simulink model "Kalman_validation"  (R2019a)
settings: Solver=VariableStepAuto  StartTime=0.0  StopTime=100.0  RelTol=1e-3
undefined symbols (not defined in the file or in its folder): DiscIntNeverNeededParam, Discrete, Time
libraries: simulink x3, ctrlSharedLib x2
settings Model: Creator=Gaming  LastModifiedBy=Gaming

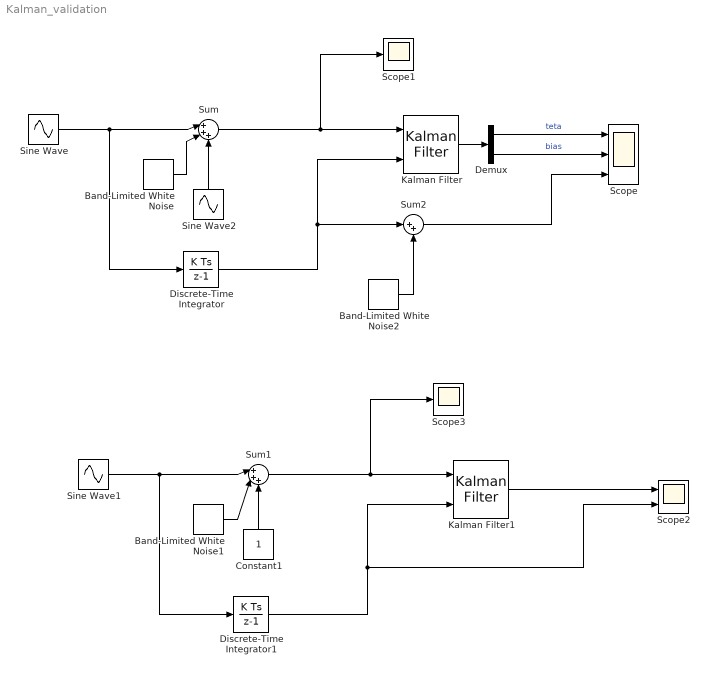
== system Kalman_validation ==
  Band-Limited White Noise : simulink/Sources/Band-Limited White Noise  Cov=[0.0001]  Ts=0.1  seed=[23341]
  Band-Limited White Noise1 : simulink/Sources/Band-Limited White Noise  Cov=[0.0001]  Ts=0.1  seed=[23341]
  Band-Limited White Noise2 : simulink/Sources/Band-Limited White Noise  Cov=[0.0001]  Ts=0.1  seed=[23341]
  Constant1 : Constant
  Demux : Demux  Outputs=2
  Discrete-Time Integrator : DiscreteIntegrator  SampleTime=-1  ICPrevOutput=DiscIntNeverNeededParam  ICPrevScaledInput=DiscIntNeverNeededParam
  Discrete-Time Integrator1 : DiscreteIntegrator  SampleTime=-1  ICPrevOutput=DiscIntNeverNeededParam  ICPrevScaledInput=DiscIntNeverNeededParam
  Kalman Filter : ctrlSharedLib/Kalman Filter  TimeDomain=Discrete-Time  UseCurrentEstimator=on  ModelSource=LTI State-Space Variable  ModelSourceVariable=ALFA  A=0.95*eye(2)  B=eye(2)  C=eye(2)  D=zeros(2)  NumberOfStates=2  NumberOfInputs=2  NumberOfOutputs=2  InitialEstimateSource=Dialog  X0=[0,;0]  P0=10  UseK=off  UseGH=off  NumberOfProcessNoiseInputs=2  G=1  TimeInvariantG=on  H=0  TimeInvariantH=on  Q=1000  TimeInvariantQ=on  R=1  TimeInvariantR=on  N=0  TimeInvariantN=on  AddInputPort=on  AddEnablePort=off  OutputEstimatedY=off  OutputP=off  Ts=-1
      settings: SourceProductBaseCode=CT
  Kalman Filter1 : ctrlSharedLib/Kalman Filter  TimeDomain=Discrete-Time  UseCurrentEstimator=on  ModelSource=LTI State-Space Variable  ModelSourceVariable=BETA  A=0.95*eye(2)  B=eye(2)  C=eye(2)  D=zeros(2)  NumberOfStates=2  NumberOfInputs=2  NumberOfOutputs=2  InitialEstimateSource=Dialog  X0=0  P0=10  UseK=off  UseGH=off  NumberOfProcessNoiseInputs=2  G=1  TimeInvariantG=on  H=0  TimeInvariantH=on  Q=1000  TimeInvariantQ=on  R=1  TimeInvariantR=on  N=0  TimeInvariantN=on  AddInputPort=on  AddEnablePort=off  OutputEstimatedY=off  OutputP=off  Ts=-1
      settings: SourceProductBaseCode=CT
  Scope : Scope  NumInputPorts=3
  Scope1 : Scope
  Scope2 : Scope  NumInputPorts=2
  Scope3 : Scope
  Sine Wave : Sin  SineType=Sample based  Amplitude=0  Samples=100  SampleTime=0.1
  Sine Wave1 : Sin  SineType=Sample based  Amplitude=0  Samples=100  SampleTime=0.1
  Sine Wave2 : Sin  SineType=Sample based  Amplitude=0  Bias=1  Samples=100  SampleTime=0.1
  Sum : Sum  Inputs=|+++
  Sum1 : Sum  Inputs=|+++
  Sum2 : Sum  Inputs=|++
  wires:
  Kalman Filter/1 -> Demux/1
  Sine Wave/1 -> Discrete-Time Integrator/1, Sum/1
  Sum/1 -> Scope1/1, Kalman Filter/1
  Discrete-Time Integrator/1 -> Sum2/1, Kalman Filter/2
  Sine Wave2/1 -> Sum/3
  Constant1/1 -> Sum1/3
  Band-Limited White Noise1/1 -> Sum1/2
  Discrete-Time Integrator1/1 -> Scope2/2, Kalman Filter1/2
  Sine Wave1/1 -> Discrete-Time Integrator1/1, Sum1/1
  Kalman Filter1/1 -> Scope2/1
  Sum1/1 -> Scope3/1, Kalman Filter1/1
  Sum2/1 -> Scope/3
  Band-Limited White Noise2/1 -> Sum2/2
  Band-Limited White Noise/1 -> Sum/2
  Demux/1 -> Scope/1  "teta"
  Demux/2 -> Scope/2  "bias"
